simulink model "HSX_PPS_series"  (R2023b)
settings: Solver=VariableStepAuto  StartTime=0.0  StopTime=20  RelTol=1e-3
undefined symbols (not defined in the file): LHSX, Ra, RHSX
libraries: spsGroundLib x6, spsCurrentMeasurementLib x4, spsSeriesRLCBranchLib x4, spsVoltageMeasurementLib x4, spsMosfetLib x2, spsControlledVoltageSourceLib x2, spsDCMachineLib x2, spsIdealSwitchLib x2, spsDCVoltageSourceLib x1, spsPWMGenerator2LevelLib x1, sps_lib x1
settings Model: Creator=Hyeongmeen  LastModifiedBy=baik3-ad

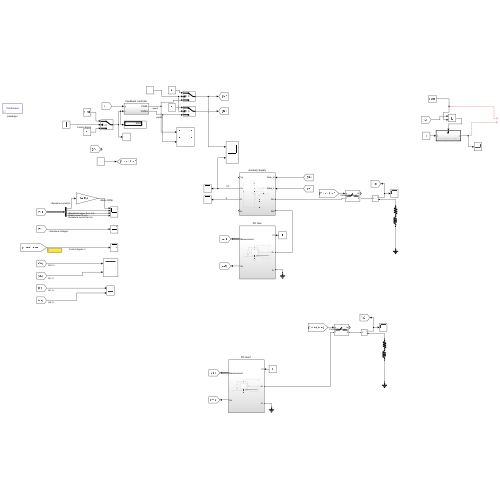
[thumbnail: Simulink's stored preview of the top-level diagram]
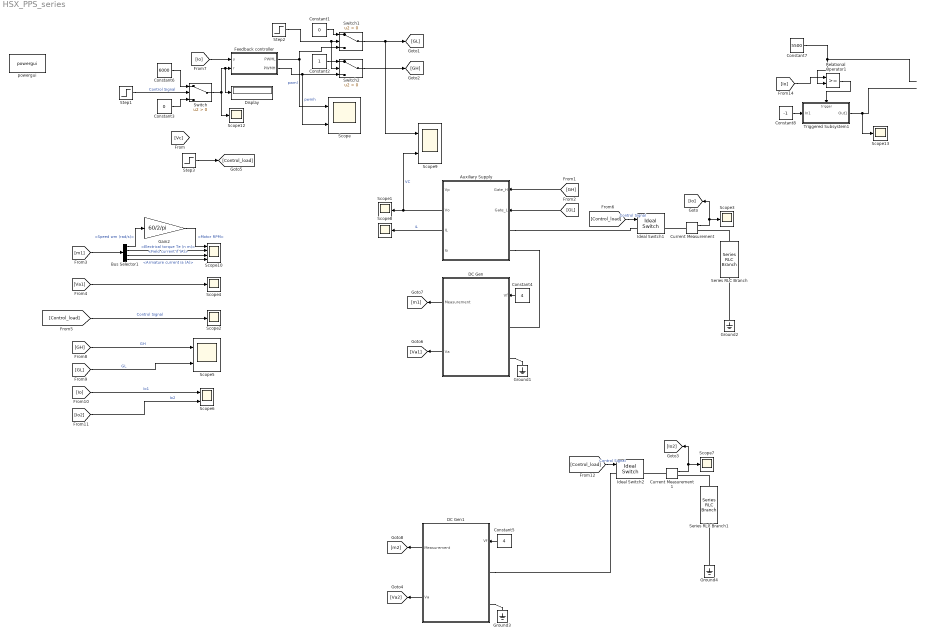
== system HSX_PPS_series ==
  Auxiliary Supply : Subsystem
  Bus Selector1 : BusSelector  OutputSignals=Speed wm (rad/s),Electrical torque Te (n m),Field current if (A),Armature current ia (A)
  Constant1 : Constant  Value=0
  Constant2 : Constant
  Constant3 : Constant  Value=0
  Constant4 : Constant  Value=4
  Constant5 : Constant  Value=4
  Constant6 : Constant  Value=6000
  Constant7 : Constant  Value=5500
  Constant8 : Constant  Value=-1
  Current Measurement : spsCurrentMeasurementLib/Current Measurement  PhasorSimulation=off  OutputType=Complex  PSBequivalent=0
  Current Measurement1 : spsCurrentMeasurementLib/Current Measurement  PhasorSimulation=off  OutputType=Complex  PSBequivalent=0
  DC Gen : Subsystem
  DC Gen1 : Subsystem
  Display : Display
  Feedback controller : Subsystem
  Gain2 : Gain  Gain=60/2/pi
  Ground{1..4} (4 alike) : spsGroundLib/Ground  LConnTagsString=a
  Ideal Switch1 : spsIdealSwitchLib/Ideal Switch  Ron=0  Lon=0  IC=0  Rs=inf  Cs=0  Measurements=on
  Ideal Switch2 : spsIdealSwitchLib/Ideal Switch  Ron=0  Lon=0  IC=0  Rs=inf  Cs=0  Measurements=on
  Relational Operator1 : RelationalOperator  OutDataTypeStr=boolean  RndMeth=Simplest  InputSameDT=off
  Scope{,5..6,9} (4 alike) : Scope  NumInputPorts=2
  Scope{1..4,7..8,12..13} (8 alike) : Scope
  Scope10 : Scope  NumInputPorts=4
  Series RLC Branch : spsSeriesRLCBranchLib/Series RLC Branch  LConnTagsString=__new0  RConnTagsString=__new0  BranchType=RL  Resistance=RHSX  Inductance=LHSX  SetiL0=off  InitialCurrent=0  Capacitance=1e-6  Setx0=off  InitialVoltage=0  Measurements=None
  Series RLC Branch1 : spsSeriesRLCBranchLib/Series RLC Branch  LConnTagsString=__new0  RConnTagsString=__new0  BranchType=RL  Resistance=RHSX  Inductance=LHSX  SetiL0=off  InitialCurrent=0  Capacitance=1e-6  Setx0=off  InitialVoltage=0  Measurements=None
  Step1 : Step  Time=10  SampleTime=0  VectorParams1D=off  ZeroCross=off
  Step2 : Step  Time=10.2  Before=1  After=0  SampleTime=0  VectorParams1D=off  ZeroCross=off
  Step3 : Step  Time=10  SampleTime=0  VectorParams1D=off  ZeroCross=off
  Switch : Switch  Criteria=u2 > Threshold  SaturateOnIntegerOverflow=off  InputSameDT=off
  Switch1 : Switch  Criteria=u2 > Threshold  SaturateOnIntegerOverflow=off  InputSameDT=off
  Switch2 : Switch  Criteria=u2 > Threshold  SaturateOnIntegerOverflow=off  InputSameDT=off
  Triggered Subsystem1 : Subsystem  TreatAsAtomicUnit=on
  powergui : sps_lib/powergui  Priority=1  SimulationMode=Continuous  SampleTime=1e-7  frequency=60  Iterations=50  frequencyindice=0  Pbase=100e6  ErrMax=1e-4  UnitsV=kV  UnitsW=MW  buscounter=0  FunctionMessages=off  echomessages=off  EnableUseOfTLC=off  CurrentSourceSwitches=off  DisableSnubberDevices=off  DisableRonSwitches=off  DisableVfSwitches=off  DisplayEquations=off  AutomaticDiscreteSolvers=off  SolverType=Tustin/Backward Euler (TBE)  Interpol=off  ExternalGateDelay=off  methode=off  Ts=100  x0status=blocks  SPID=on  SwTol=0  HookPort=off  NonlinearTolerance=1e-4  nMaxIteration=100  ContinueOnMaxIteration=off  RestoreLinks=warning  ResistiveCurrentMeasurement=off  Frange=[0:2:500]  Ylog=off  Xlog=on  ShowGrid=off  save=off  variable=ZData  structure=0  ZoomFFT=off  StartTime=0.0  cycles=1  DisplayStyle=1  fundamental=60  FreqAxis=off  MaxFrequency=1000  frequencyindicesteady=1  RmsSteady=1  display=off
  wires:
  Bus Selector1/1 -> Gain2/1  "<Speed wm (rad/s)>"
  Bus Selector1/4 -> Scope10/4  "<Armature current ia (A)>"
  Bus Selector1/2 -> Scope10/2  "<Electrical torque Te (n m)>"
  Gain2/1 -> Scope10/1  "<Motor RPM>"
  Bus Selector1/3 -> Scope10/3  "<Field current if (A)>"
  [m1] -> Bus Selector1/1
  Step3/1 -> [Control_load]
  Step2/1 -> Switch2/2, Switch1/2
  Feedback controller/2(PWMH) -> Switch2/3, Scope/2  "pwmh"
  Switch/1 -> Scope12/1, Display/1, Feedback controller/2(r)
  Feedback controller/1(PWML) -> Switch1/3, Scope/1  "pwml"
  [Io] -> Feedback controller/1(y)
  Constant1/1 -> Switch1/1
  Constant2/1 -> Switch2/1
  [Control_load] -> Scope2/1  "Control Signal"
  [Va1] -> Scope4/1
  DC Gen/1(Measurement) -> [m1]
  Constant4/1 -> DC Gen/1(Vf)
  DC Gen/2(Va) -> [Va1]
  Switch2/1 -> [GH]
  Switch1/1 -> Scope9/1, [GL]
  [GH] -> Auxiliary Supply/1(Gate_H)
  [GL] -> Auxiliary Supply/2(Gate_L)
  Auxiliary Supply/2(Vo) -> Scope9/2, Scope1/1  "VC"
  [Control_load] -> Ideal Switch1/1  "Control Signal"
  Current Measurement/1 -> [Io], Scope3/1
  Constant3/1 -> Switch/3
  [GH] -> Scope5/1  "GH"
  [GL] -> Scope5/2  "GL"
  [Control_load] -> Ideal Switch2/1  "Control Signal"
  DC Gen1/2(Va) -> [Va2]
  Constant5/1 -> DC Gen1/1(Vf)
  DC Gen1/1(Measurement) -> [m2]
  Current Measurement1/1 -> [Io2], Scope7/1
  [Io] -> Scope6/1  "Io1"
  [Io2] -> Scope6/2  "Io2"
  Auxiliary Supply/3(IL) -> Scope8/1  "iL"
  Constant8/1 -> Triggered Subsystem1/1(In1)
  [Io] -> Relational Operator1/1
  Constant7/1 -> Relational Operator1/2
  Relational Operator1/1 -> Triggered Subsystem1/Trigger
  Triggered Subsystem1/1(Out1) -> Scope13/1
  Step1/1 -> Switch/2  "Control Signal"
  Constant6/1 -> Switch/1
  connections:
  DC Gen/LConn2 -- Ground1/LConn1
  Auxiliary Supply/LConn2 -- DC Gen/LConn1
  Auxiliary Supply/LConn1 -- Ideal Switch1/LConn1
  Ground2/LConn1 -- Series RLC Branch/RConn1
  Current Measurement/LConn1 -- Ideal Switch1/RConn1
  Series RLC Branch/LConn1 -- Current Measurement/RConn1
  DC Gen1/LConn2 -- Ground3/LConn1
  DC Gen1/LConn1 -- Ideal Switch2/LConn1
  Series RLC Branch1/LConn1 -- Current Measurement1/RConn1
  Current Measurement1/LConn1 -- Ideal Switch2/RConn1
  Ground4/LConn1 -- Series RLC Branch1/RConn1

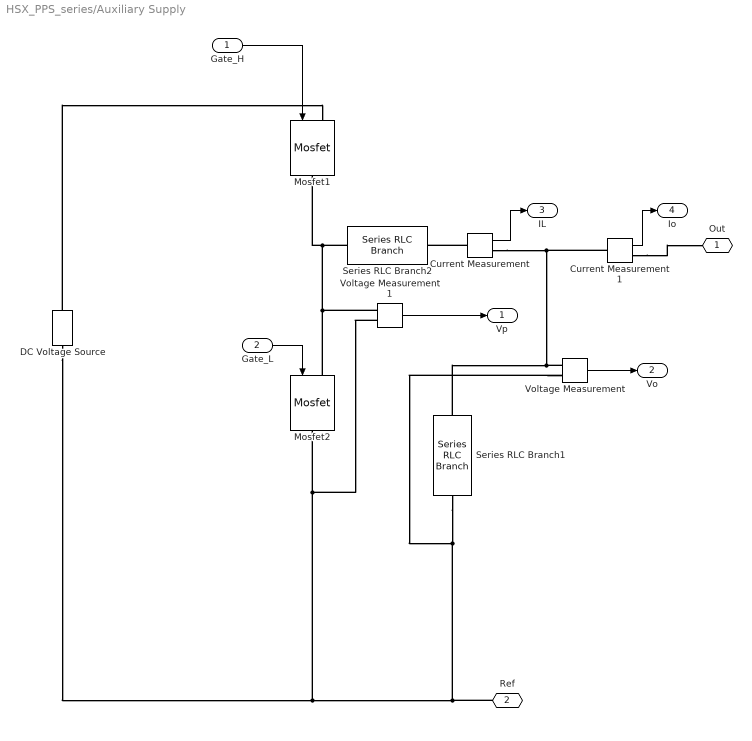
== system HSX_PPS_series/Auxiliary Supply ==
  Gate_H : Inport
  Gate_L : Inport  Port=2
  Current Measurement : spsCurrentMeasurementLib/Current Measurement  PhasorSimulation=off  OutputType=Complex  PSBequivalent=0
  Current Measurement1 : spsCurrentMeasurementLib/Current Measurement  PhasorSimulation=off  OutputType=Complex  PSBequivalent=0
  DC Voltage Source : spsDCVoltageSourceLib/DC Voltage Source  Amplitude=1000  Measurements=None
  Mosfet1 : spsMosfetLib/Mosfet  Ron=0.1  Lon=0  Rd=0.01  Vfd=0.8  IC=0  Rs=1e5  Cs=inf  Measurements=off
  Mosfet2 : spsMosfetLib/Mosfet  Ron=0.1  Lon=0  Rd=0.01  Vfd=0.8  IC=0  Rs=1e5  Cs=inf  Measurements=off
  Series RLC Branch1 : spsSeriesRLCBranchLib/Series RLC Branch  LConnTagsString=__new0  RConnTagsString=__new0  BranchType=C  Resistance=0.09  Inductance=0.02  SetiL0=off  InitialCurrent=0  Capacitance=1e-3  Setx0=on  InitialVoltage=0  Measurements=None
  Series RLC Branch2 : spsSeriesRLCBranchLib/Series RLC Branch  LConnTagsString=__new0  RConnTagsString=__new0  BranchType=L  Resistance=0.09  Inductance=0.0001  SetiL0=off  InitialCurrent=0  Capacitance=1e-1  Setx0=off  InitialVoltage=0  Measurements=None
  Voltage Measurement : spsVoltageMeasurementLib/Voltage Measurement  PhasorSimulation=off  OutputType=Complex  PSBequivalent=0
  Voltage Measurement1 : spsVoltageMeasurementLib/Voltage Measurement  PhasorSimulation=off  OutputType=Complex  PSBequivalent=0
  Out : PMIOPort  Side=Left
  Ref : PMIOPort  Port=2  Side=Left
  Vp : Outport
  Vo : Outport  Port=2
  IL : Outport  Port=3
  Io : Outport  Port=4
  wires:
  Gate_L/1 -> Mosfet2/1
  Gate_H/1 -> Mosfet1/1
  Voltage Measurement1/1 -> Vp/1
  Voltage Measurement/1 -> Vo/1
  Current Measurement/1 -> IL/1
  Current Measurement1/1 -> Io/1
  connections:
  Mosfet1/RConn1 -- Series RLC Branch2/LConn1 -- Voltage Measurement1/LConn1 -- Mosfet2/LConn1
  Voltage Measurement/LConn1 -- Current Measurement1/LConn1 -- Current Measurement/RConn1 -- Series RLC Branch1/LConn1
  Series RLC Branch1/RConn1 -- Ref/RConn1 -- DC Voltage Source/LConn1 -- Voltage Measurement1/LConn2 -- Mosfet2/RConn1 -- Voltage Measurement/LConn2
  DC Voltage Source/RConn1 -- Mosfet1/LConn1
  Current Measurement/LConn1 -- Series RLC Branch2/RConn1
  Current Measurement1/RConn1 -- Out/RConn1

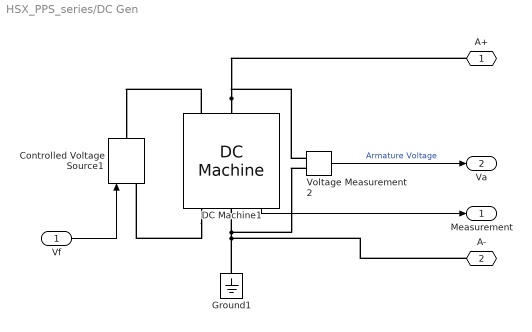
== system HSX_PPS_series/DC Gen ==
  Vf : Inport
  Controlled Voltage Source1 : spsControlledVoltageSourceLib/Controlled Voltage Source  Initialize=on  Source_Type=DC  Amplitude=0  Phase=0  Frequency=0  Measurements=Voltage
  DC Machine1 : spsDCMachineLib/DC Machine  PresetModel=No  MechanicalLoad=Torque TL  FieldType=Wound  ShowDetailedParameters=on  MeasurementBus=off  RLa="[Ra  0.002]"  RLf=[0.0054 0.0125]  Laf=Laf  MachineConstant=Torque constant (N.m/A)  Ke=1.8  Kt=1.8  J=137  Bm=0  Tf=0  w0=w_initial  Ifinit=0  TsPowergui=0  TsBlock=-1
  Ground1 : spsGroundLib/Ground  LConnTagsString=a
  Voltage Measurement2 : spsVoltageMeasurementLib/Voltage Measurement  PhasorSimulation=off  OutputType=Complex  PSBequivalent=0
  A+ : PMIOPort  Side=Left
  A- : PMIOPort  Port=2  Side=Left
  Measurement : Outport
  Va : Outport  Port=2
  wires:
  DC Machine1/1 -> Measurement/1
  Vf/1 -> Controlled Voltage Source1/1
  Voltage Measurement2/1 -> Va/1  "Armature Voltage"
  connections:
  DC Machine1/LConn1 -- Voltage Measurement2/LConn1 -- A+/RConn1
  Ground1/LConn1 -- DC Machine1/RConn1 -- Voltage Measurement2/LConn2 -- A-/RConn1
  DC Machine1/LConn2 -- Controlled Voltage Source1/RConn1
  DC Machine1/RConn2 -- Controlled Voltage Source1/LConn1

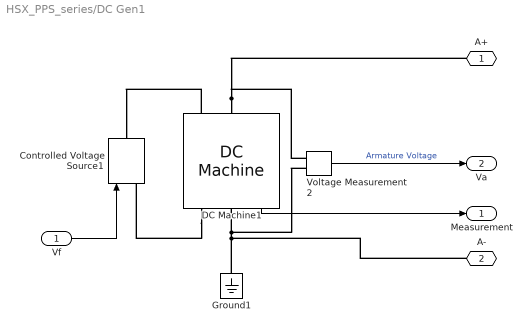
== system HSX_PPS_series/DC Gen1 ==
  Vf : Inport
  Controlled Voltage Source1 : spsControlledVoltageSourceLib/Controlled Voltage Source  Initialize=on  Source_Type=DC  Amplitude=0  Phase=0  Frequency=0  Measurements=Voltage
  DC Machine1 : spsDCMachineLib/DC Machine  PresetModel=No  MechanicalLoad=Torque TL  FieldType=Wound  ShowDetailedParameters=on  MeasurementBus=off  RLa="[Ra  0.002]"  RLf=[0.0054 0.0125]  Laf=Laf  MachineConstant=Torque constant (N.m/A)  Ke=1.8  Kt=1.8  J=137  Bm=0  Tf=0  w0=w_initial  Ifinit=0  TsPowergui=0  TsBlock=-1
  Ground1 : spsGroundLib/Ground  LConnTagsString=a
  Voltage Measurement2 : spsVoltageMeasurementLib/Voltage Measurement  PhasorSimulation=off  OutputType=Complex  PSBequivalent=0
  A+ : PMIOPort  Side=Left
  A- : PMIOPort  Port=2  Side=Left
  Measurement : Outport
  Va : Outport  Port=2
  wires:
  DC Machine1/1 -> Measurement/1
  Vf/1 -> Controlled Voltage Source1/1
  Voltage Measurement2/1 -> Va/1  "Armature Voltage"
  connections:
  DC Machine1/LConn1 -- Voltage Measurement2/LConn1 -- A+/RConn1
  Ground1/LConn1 -- DC Machine1/RConn1 -- Voltage Measurement2/LConn2 -- A-/RConn1
  DC Machine1/LConn2 -- Controlled Voltage Source1/RConn1
  DC Machine1/RConn2 -- Controlled Voltage Source1/LConn1

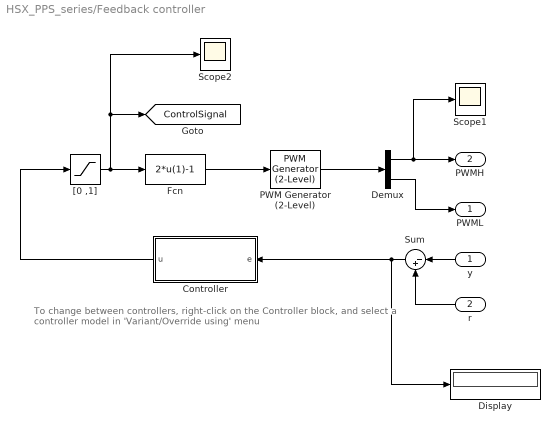
== system HSX_PPS_series/Feedback controller ==
  note: To change between controllers, right-click on the Controller block,
      | and select a controller model in 'Variant/Override using' menu
  y : Inport
  r : Inport  Port=2
  Controller : Subsystem  Variant=on  VariantControlMode=label  LabelModeActiveChoice=Variant1
      settings: AttributesFormatString=%<BlockChoice>
  Demux : Demux  Outputs=2
  Display : Display
  Fcn : Fcn  Expr=2*u(1)-1
  PWM Generator (2-Level) : spsPWMGenerator2LevelLib/PWM Generator (2-Level)  ModulatorType=Single-phase half-bridge (2 pulses)  ModulatorMode=Unsynchronized  Fc=10000  Pc=90  nF=27  MinMax="[ -1  1 ]"  SamplingTechnique=Natural  ModulatingSignals=off  m=0.8  Freq=60  Phase=0  Ts=0  ShowCarrierOutport=off
  Scope1 : Scope
  Scope2 : Scope
  Sum : Sum  Inputs=|-+  InputSameDT=on  SaturateOnIntegerOverflow=on  OutDataTypeStr=Inherit: Same as first input
  "[0 ,1]" : Saturate  UpperLimit=1  LowerLimit=0
  PWML : Outport  VectorParamsAs1DForOutWhenUnconnected=off
  PWMH : Outport  Port=2  VectorParamsAs1DForOutWhenUnconnected=off
  tag scope: ControlSignal=global
  wires:
  Controller/1(u) -> "[0 ,1]"/1
  Sum/1 -> Controller/1(e), Display/1
  y/1 -> Sum/1
  r/1 -> Sum/2
  "[0 ,1]"/1 -> Fcn/1, Scope2/1, [ControlSignal]
  Fcn/1 -> PWM Generator (2-Level)/1
  PWM Generator (2-Level)/1 -> Demux/1
  Demux/1 -> Scope1/1, PWMH/1
  Demux/2 -> PWML/1

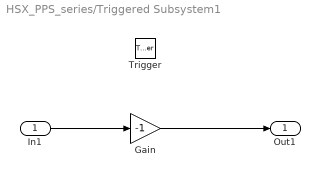
== system HSX_PPS_series/Triggered Subsystem1 ==
  In1 : Inport
  Trigger : TriggerPort  VariantControl=(inherit)
  Gain : Gain  Gain=-1
  Out1 : Outport
  wires:
  In1/1 -> Gain/1
  Gain/1 -> Out1/1

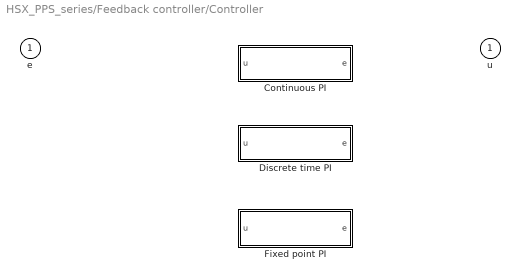
== system HSX_PPS_series/Feedback controller/Controller ==
  e : Inport
  Continuous PI : Subsystem  VariantControl=Variant1
  Discrete time PI : Subsystem  VariantControl=Variant2
  Fixed point PI : Subsystem  MinMaxOverflowLogging=MinMaxAndOverflow  VariantControl=Variant3
  u : Outport  VectorParamsAs1DForOutWhenUnconnected=off

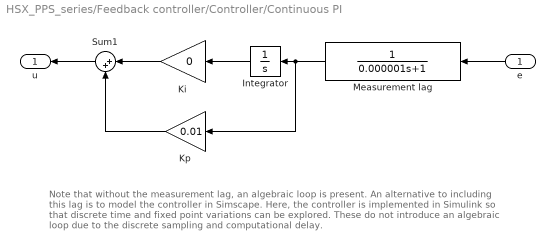
== system HSX_PPS_series/Feedback controller/Controller/Continuous PI ==
  note: Note that without the measurement lag, an algebraic loop is present. An alternative to
      | including this lag is to model the controller in Simscape. Here, the controller is implemented
      | in Simulink so that discrete time and fixed point variations can be explored. These do not
      | introduce an algebraic loop due to the discrete sampling and computational delay.
  e : Inport
  Integrator : Integrator
  Ki : Gain  Gain=0
  Kp : Gain  Gain=0.01
  Measurement lag : TransferFcn  Denominator=[0.000001 1]
  Sum1 : Sum  Inputs=|++  InputSameDT=on  SaturateOnIntegerOverflow=on  OutDataTypeStr=Inherit: Same as first input
  u : Outport  VectorParamsAs1DForOutWhenUnconnected=off
  wires:
  Measurement lag/1 -> Kp/1, Integrator/1
  Ki/1 -> Sum1/1
  Sum1/1 -> u/1
  Kp/1 -> Sum1/2
  Integrator/1 -> Ki/1
  e/1 -> Measurement lag/1

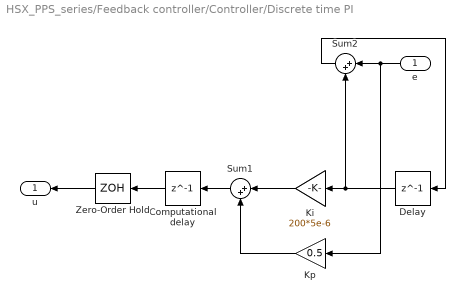
== system HSX_PPS_series/Feedback controller/Controller/Discrete time PI ==
  e : Inport
  Computational delay : Delay  DelayLength=1  SampleTime=5e-6
  Delay : Delay  DelayLength=1  SampleTime=5e-6
  Ki : Gain  Gain=200*5e-6
  Kp : Gain  Gain=0.5
  Sum1 : Sum  Inputs=|++  InputSameDT=on  SaturateOnIntegerOverflow=on  OutDataTypeStr=Inherit: Same as first input
  Sum2 : Sum  Inputs=|++  InputSameDT=on  SaturateOnIntegerOverflow=on  OutDataTypeStr=Inherit: Same as first input
  Zero-Order Hold : ZeroOrderHold  SampleTime=5e-6
  u : Outport  VectorParamsAs1DForOutWhenUnconnected=off
  wires:
  Ki/1 -> Sum1/1
  Sum2/1 -> Delay/1
  Delay/1 -> Ki/1, Sum2/2
  Kp/1 -> Sum1/2
  Sum1/1 -> Computational delay/1
  e/1 -> Kp/1, Sum2/1
  Zero-Order Hold/1 -> u/1
  Computational delay/1 -> Zero-Order Hold/1

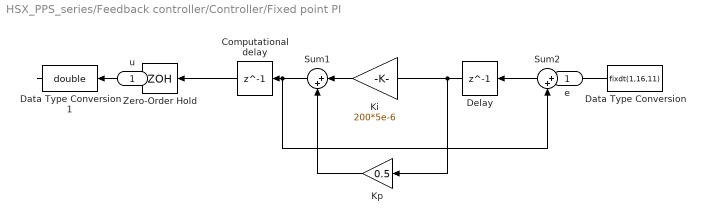
== system HSX_PPS_series/Feedback controller/Controller/Fixed point PI ==
  e : Inport
  Computational delay : Delay  DelayLength=1  SampleTime=5e-6
  Data Type Conversion : DataTypeConversion  OutDataTypeStr=fixdt(1,16,11)  RndMeth=Nearest  SaturateOnIntegerOverflow=off
  Data Type Conversion1 : DataTypeConversion  OutDataTypeStr=double  RndMeth=Nearest  SaturateOnIntegerOverflow=off
  Delay : Delay  DelayLength=1  SampleTime=5e-6
  Ki : Gain  Gain=200*5e-6  OutDataTypeStr=fixdt(1,16,13)  RndMeth=Nearest
  Kp : Gain  Gain=0.5  OutDataTypeStr=fixdt(1,16,9)  RndMeth=Nearest
  Sum1 : Sum  Inputs=|++  SaturateOnIntegerOverflow=on
  Sum2 : Sum  Inputs=|++  InputSameDT=on  SaturateOnIntegerOverflow=on  OutDataTypeStr=Inherit: Same as first input
  Zero-Order Hold : ZeroOrderHold  SampleTime=5e-6
  u : Outport  VectorParamsAs1DForOutWhenUnconnected=off
  wires:
  Ki/1 -> Sum1/1
  Data Type Conversion1/1 -> u/1
  Data Type Conversion/1 -> Sum2/1, Kp/1
  Sum1/1 -> Computational delay/1
  Kp/1 -> Sum1/2
  e/1 -> Data Type Conversion/1
  Delay/1 -> Ki/1, Sum2/2
  Sum2/1 -> Delay/1
  Computational delay/1 -> Zero-Order Hold/1
  Zero-Order Hold/1 -> Data Type Conversion1/1
